simulink model "HIL_Testing_SW_amantest"  (Simulink 7.5)
settings: Solver=ode1  StartTime=0.0  StopTime=Inf  FixedStep=0.001  RelTol=1e-3
PostLoadFcn:
  | , if any(exist('dsrtsu_mdlpostloadfcn', 'file') == [2, 3, 6]), try dsrtsu_mdlpostloadfcn('Execute', bdroot); catch fprintf('Error in PostLoadFcn (dsrtsu_mdlpostloadfcn) for model "%s":\n %s\n', bdroot, lasterr); end, end,
undefined symbols (not defined in the file): CeBSER_Cnt_NumTempAxisPts, ChargeCord, ChargeCord_Control, ChargeToSOCCurr, ChrgCurrLim, CrntSens1Fine, CS_SOCSetPt, CyclerMaxChrgPwr, CyclerMaxDschrgPwr, deltaAhr, Drive_1, Drive_10, Drive_11, Drive_12, Drive_13, Drive_14, Drive_15, Drive_16, Drive_17, Drive_18, Drive_19, Drive_2, Drive_20, Drive_21, Drive_22, Drive_23, Drive_24, Drive_25, Drive_26, Drive_27, Drive_28, Drive_29, Drive_3, Drive_30, Drive_31, Drive_32, Drive_33, Drive_34, Drive_35, Drive_36, Drive_37, Drive_38, Drive_39, Drive_4, Drive_40, Drive_41, Drive_42, Drive_43, Drive_44, Drive_45, Drive_46, Drive_47, Drive_48, Drive_49, Drive_5, Drive_50, Drive_51, Drive_6, Drive_7, Drive_8 ... (+50)
libraries: simulink x129, rtican x50, rti2211sailib x5, rti2211serlib x5, rti2202miolib x3
(part 5 of 23)

== system HIL_Testing_SW_amantest/RX/Read EREV ==
  Enable : EnablePort
  Read HVEM : Subsystem
  Read PTEX : Subsystem
  LT_PwrDschLmt : Outport  OutDataType=sfix(16)  OutScaling=2^0
  LT_PwrChgLmt : Outport  Port=2  OutDataType=sfix(16)  OutScaling=2^0
  SOC : Outport  Port=3  OutDataType=sfix(16)  OutScaling=2^0
  SumOfCells : Outport  Port=4  OutDataType=sfix(16)  OutScaling=2^0
  MinCell : Outport  Port=5  OutDataType=sfix(16)  OutScaling=2^0
  MaxCell : Outport  Port=6  OutDataType=sfix(16)  OutScaling=2^0
  MinSectionVoltage : Outport  Port=7  OutDataType=sfix(16)  OutScaling=2^0
  HVCntctrStat : Outport  Port=8  OutDataType=sfix(16)  OutScaling=2^0
  PackCurrent : Outport  Port=9  OutDataType=sfix(16)  OutScaling=2^0
  PackVoltage : Outport  Port=10  OutDataType=sfix(16)  OutScaling=2^0
  BatTemp : Outport  Port=11  OutDataType=sfix(16)  OutScaling=2^0
  HVBatVltUpLmt_CAN : Outport  Port=12  OutDataType=sfix(16)  OutScaling=2^0
  HVBatVltLwLmt_CAN : Outport  Port=13  OutDataType=sfix(16)  OutScaling=2^0
  HVBatStOfChrgMin_CAN : Outport  Port=14  OutDataType=sfix(16)  OutScaling=2^0
  HVBatCrntLwLmt_CAN : Outport  Port=15  OutDataType=sfix(16)  OutScaling=2^0
  HVBatCrntUpLmt_CAN : Outport  Port=16  OutDataType=sfix(16)  OutScaling=2^0
  wires:
  Read PTEX/1(LT_PwrDschLmt) -> LT_PwrDschLmt/1
  Read PTEX/2(LT_PwrChgLmt) -> LT_PwrChgLmt/1
  Read PTEX/3(SOC) -> SOC/1
  Read HVEM/1(SumOfCells) -> SumOfCells/1
  Read HVEM/2(MinCell) -> MinCell/1
  Read HVEM/3(MaxCell) -> MaxCell/1
  Read HVEM/4(MinSectionVoltage) -> MinSectionVoltage/1
  Read HVEM/5(HVCntctrStat) -> HVCntctrStat/1
  Read HVEM/6(PackCurrent) -> PackCurrent/1
  Read HVEM/7(PackVoltage) -> PackVoltage/1
  Read HVEM/8(BatTemp) -> BatTemp/1
  Read PTEX/4(HVBatVltUpLmt_CAN) -> HVBatVltUpLmt_CAN/1
  Read PTEX/5(HVBatVltLwLmt_CAN) -> HVBatVltLwLmt_CAN/1
  Read PTEX/6(HVBatStOfChrgMin_CAN) -> HVBatStOfChrgMin_CAN/1
  Read PTEX/7(HVBatCrntLwLmt_CAN) -> HVBatCrntLwLmt_CAN/1
  Read PTEX/8(HVBatCrntUpLmt_CAN) -> HVBatCrntUpLmt_CAN/1

== system HIL_Testing_SW_amantest/TX/Chamber ==
  BatTemp : Inport  OutDataType=fixdt(1, 16)  OutScaling=2^0
  SetChamberT_ToBatTemp : Inport  Port=2  OutDataType=fixdt(1, 16)  OutScaling=2^0
  ChamberT_SwitchSlct : Subsystem  TreatAsAtomicUnit=on
  Multiport Switch : MultiPortSwitch  Inputs=39  zeroidx=off  OutDataTypeMode=uint8  OutDataType=fixdt(1, 16)  OutScaling=2^0  OutDataTypeStr=uint8
  SendTxToChamber : Subsystem  TreatAsAtomicUnit=on
  SetChamberTo10C : Constant  Value=[1 6 0 60 0 100 72 45]  OutDataTypeMode=uint8  OutDataType=fixdt(1, 16)  OutScaling=2^0  OutDataTypeStr=uint8
  SetChamberTo12p5C : Constant  Value=[1 6 0 60 0 125 137 231]  OutDataTypeMode=uint8  OutDataType=fixdt(1, 16)  OutScaling=2^0  OutDataTypeStr=uint8
  SetChamberTo15C : Constant  Value=[1 6 0 60 0 150 201 168]  OutDataTypeMode=uint8  OutDataType=fixdt(1, 16)  OutScaling=2^0  OutDataTypeStr=uint8
  SetChamberTo17p5C : Constant  Value=[1 6 0 60 0 175 9 186]  OutDataTypeMode=uint8  OutDataType=fixdt(1, 16)  OutScaling=2^0  OutDataTypeStr=uint8
  SetChamberTo20C : Constant  Value=[1 6 0 60 0 200 72 80]  OutDataTypeMode=uint8  OutDataType=fixdt(1, 16)  OutScaling=2^0  OutDataTypeStr=uint8
  SetChamberTo22p5C : Constant  Value=[1 6 0 60 0 225 137 142]  OutDataTypeMode=uint8  OutDataType=fixdt(1, 16)  OutScaling=2^0  OutDataTypeStr=uint8
  SetChamberTo25C : Constant  Value=[1 6 0 60 0 250 201 133]  OutDataTypeMode=uint8  OutDataType=fixdt(1, 16)  OutScaling=2^0  OutDataTypeStr=uint8
  SetChamberTo27p5C : Constant  Value=[1 6 0 60 1 19 9 155]  OutDataTypeMode=uint8  OutDataType=fixdt(1, 16)  OutScaling=2^0  OutDataTypeStr=uint8
  SetChamberTo2p5C : Constant  Value=[1 6 0 60 0 25 136 12]  OutDataTypeMode=uint8  OutDataType=fixdt(1, 16)  OutScaling=2^0  OutDataTypeStr=uint8
  SetChamberTo30C : Constant  Value=[1 6 0 60 1 44 73 139]  OutDataTypeMode=uint8  OutDataType=fixdt(1, 16)  OutScaling=2^0  OutDataTypeStr=uint8
  SetChamberTo32p5C : Constant  Value=[1 6 0 60 1 69 137 165]  OutDataTypeMode=uint8  OutDataType=fixdt(1, 16)  OutScaling=2^0  OutDataTypeStr=uint8
  SetChamberTo35C : Constant  Value=[1 6 0 60 1 94 201 174]  OutDataTypeMode=uint8  OutDataType=fixdt(1, 16)  OutScaling=2^0  OutDataTypeStr=uint8
  SetChamberTo37p5C : Constant  Value=[1 6 0 60 1 119 8 112]  OutDataTypeMode=uint8  OutDataType=fixdt(1, 16)  OutScaling=2^0  OutDataTypeStr=uint8
  SetChamberTo40C : Constant  Value=[1 6 0 60 1 144 72 58]  OutDataTypeMode=uint8  OutDataType=fixdt(1, 16)  OutScaling=2^0  OutDataTypeStr=uint8
  SetChamberTo42p5C : Constant  Value=[1 6 0 60 1 169 136 40]  OutDataTypeMode=uint8  OutDataType=fixdt(1, 16)  OutScaling=2^0  OutDataTypeStr=uint8
  SetChamberTo45C : Constant  Value=[1 6 0 60 1 194 201 199]  OutDataTypeMode=uint8  OutDataType=fixdt(1, 16)  OutScaling=2^0  OutDataTypeStr=uint8
  SetChamberTo47p5C : Constant  Value=[1 6 0 60 1 219 8 13]  OutDataTypeMode=uint8  OutDataType=fixdt(1, 16)  OutScaling=2^0  OutDataTypeStr=uint8
  SetChamberTo50C : Constant  Value=[1 6 0 60 1 244 73 209]  OutDataTypeMode=uint8  OutDataType=fixdt(1, 16)  OutScaling=2^0  OutDataTypeStr=uint8
  SetChamberTo52p5C : Constant  Value=[1 6 0 60 2 13 137 99]  OutDataTypeMode=uint8  OutDataType=fixdt(1, 16)  OutScaling=2^0  OutDataTypeStr=uint8
  SetChamberTo55C : Constant  Value=[1 6 0 60 2 38 201 124]  OutDataTypeMode=uint8  OutDataType=fixdt(1, 16)  OutScaling=2^0  OutDataTypeStr=uint8
  SetChamberTo57p5C : Constant  Value=[1 6 0 60 2 63 8 182]  OutDataTypeMode=uint8  OutDataType=fixdt(1, 16)  OutScaling=2^0  OutDataTypeStr=uint8
  SetChamberTo5C : Constant  Value=[1 6 0 60 0 50 200 19]  OutDataTypeMode=uint8  OutDataType=fixdt(1, 16)  OutScaling=2^0  OutDataTypeStr=uint8
  SetChamberTo60C : Constant  Value=[1 6 0 60 2 88 73 92]  OutDataTypeMode=uint8  OutDataType=fixdt(1, 16)  OutScaling=2^0  OutDataTypeStr=uint8
  SetChamberTo62p5C : Constant  Value=[1 6 0 60 2 113 136 130]  OutDataTypeMode=uint8  OutDataType=fixdt(1, 16)  OutScaling=2^0  OutDataTypeStr=uint8
  SetChamberTo65C : Constant  Value="[1 6 0 60 2  138 201 1]"  OutDataTypeMode=uint8  OutDataType=fixdt(1, 16)  OutScaling=2^0  OutDataTypeStr=uint8
  SetChamberTo7p5C : Constant  Value=[1 6 0 60 0 75 9 241]  OutDataTypeMode=uint8  OutDataType=fixdt(1, 16)  OutScaling=2^0  OutDataTypeStr=uint8
  SetChamberToMinus10C : Constant  Value=[1 6 0 60 255 156 8 95]  OutDataTypeMode=uint8  OutDataType=fixdt(1, 16)  OutScaling=2^0  OutDataTypeStr=uint8
  SetChamberToMinus12p5C : Constant  Value=[1 6 0 60 255 131 73 151]  OutDataTypeMode=uint8  OutDataType=fixdt(1, 16)  OutScaling=2^0  OutDataTypeStr=uint8
  SetChamberToMinus15C : Constant  Value=[1 6 0 60 255 106 136 25]  OutDataTypeMode=uint8  OutDataType=fixdt(1, 16)  OutScaling=2^0  OutDataTypeStr=uint8
  SetChamberToMinus17p5C : Constant  Value=[1 6 0 60 255 81 201 202]  OutDataTypeMode=uint8  OutDataType=fixdt(1, 16)  OutScaling=2^0  OutDataTypeStr=uint8
  SetChamberToMinus20C : Constant  Value=[1 6 0 60 255 56 9 228]  OutDataTypeMode=uint8  OutDataType=fixdt(1, 16)  OutScaling=2^0  OutDataTypeStr=uint8
  SetChamberToMinus22p5C : Constant  Value=[1 6 0 60 255 31 73 254]  OutDataTypeMode=uint8  OutDataType=fixdt(1, 16)  OutScaling=2^0  OutDataTypeStr=uint8
  SetChamberToMinus25C : Constant  Value=[1 6 0 60 255 6 136 52]  OutDataTypeMode=uint8  OutDataType=fixdt(1, 16)  OutScaling=2^0  OutDataTypeStr=uint8
  SetChamberToMinus27p5C : Constant  Value=[1 6 0 60 254 237 201 235]  OutDataTypeMode=uint8  OutDataType=fixdt(1, 16)  OutScaling=2^0  OutDataTypeStr=uint8
  SetChamberToMinus2p5C : Constant  Value=[1 6 0 60 255 231 72 124]  OutDataTypeMode=uint8  OutDataType=fixdt(1, 16)  OutScaling=2^0  OutDataTypeStr=uint8
  SetChamberToMinus30C : Constant  Value=[1 6 0 60 254 212 9 249]  OutDataTypeMode=uint8  OutDataType=fixdt(1, 16)  OutScaling=2^0  OutDataTypeStr=uint8
  SetChamberToMinus5C : Constant  Value=[1 6 0 60 255 206 137 162]  OutDataTypeMode=uint8  OutDataType=fixdt(1, 16)  OutScaling=2^0  OutDataTypeStr=uint8
  SetChamberToMinus7p5C : Constant  Value=[1 6 0 60 255 181 201 129]  OutDataTypeMode=uint8  OutDataType=fixdt(1, 16)  OutScaling=2^0  OutDataTypeStr=uint8
  SetChamberToZeroC : Constant  Value=[1 6 0 60 0 0 73 198]  OutDataTypeMode=uint8  OutDataType=fixdt(1, 16)  OutScaling=2^0  OutDataTypeStr=uint8
  Trigger_200ms : Subsystem  TreatAsAtomicUnit=on
      settings: CopyFcn=breaklink(gcb)
      mask Type: EnabledFunctionCall
      mask Description:
      | Execute a function-call subsystem at an inherited rate if enabled.
      | 
      | Demux the block's output to execute multiple function-call subsystems in a prescribed order.  The system connected to first demux port is executed first, the system connected to second demux port is executed second, and so on.
      mask Help: web(char(which([char(get_param(gcb,'MaskType')),'.html'])));
      mask Display: disp('f()')
  Trigger_200ms2 : Subsystem  TreatAsAtomicUnit=on
      settings: CopyFcn=breaklink(gcb)
      mask Type: EnabledFunctionCall
      mask Description:
      | Execute a function-call subsystem at an inherited rate if enabled.
      | 
      | Demux the block's output to execute multiple function-call subsystems in a prescribed order.  The system connected to first demux port is executed first, the system connected to second demux port is executed second, and so on.
      mask Help: web(char(which([char(get_param(gcb,'MaskType')),'.html'])));
      mask Display: disp('f()')
  wires:
  Multiport Switch/1 -> SendTxToChamber/1(ChamberTempCommand)
  Trigger_200ms2/1(Output Parameter) -> ChamberT_SwitchSlct/Trigger
  Trigger_200ms/1(Output Parameter) -> SendTxToChamber/Trigger  "TriggerMe"
  SetChamberToMinus30C/1 -> Multiport Switch/2
  SetChamberToMinus27p5C/1 -> Multiport Switch/3
  SetChamberToMinus25C/1 -> Multiport Switch/4
  SetChamberToMinus22p5C/1 -> Multiport Switch/5
  SetChamberToMinus20C/1 -> Multiport Switch/6
  SetChamberToMinus17p5C/1 -> Multiport Switch/7
  SetChamberToMinus15C/1 -> Multiport Switch/8
  SetChamberToMinus12p5C/1 -> Multiport Switch/9
  SetChamberToMinus10C/1 -> Multiport Switch/10
  SetChamberToMinus7p5C/1 -> Multiport Switch/11
  SetChamberToMinus5C/1 -> Multiport Switch/12
  SetChamberToMinus2p5C/1 -> Multiport Switch/13
  SetChamberToZeroC/1 -> Multiport Switch/14
  SetChamberTo2p5C/1 -> Multiport Switch/15
  SetChamberTo5C/1 -> Multiport Switch/16
  SetChamberTo7p5C/1 -> Multiport Switch/17
  SetChamberTo10C/1 -> Multiport Switch/18
  SetChamberTo12p5C/1 -> Multiport Switch/19
  SetChamberTo15C/1 -> Multiport Switch/20
  SetChamberTo17p5C/1 -> Multiport Switch/21
  SetChamberTo20C/1 -> Multiport Switch/22
  SetChamberTo22p5C/1 -> Multiport Switch/23
  SetChamberTo25C/1 -> Multiport Switch/24
  SetChamberTo27p5C/1 -> Multiport Switch/25
  SetChamberTo30C/1 -> Multiport Switch/26
  SetChamberTo32p5C/1 -> Multiport Switch/27
  SetChamberTo35C/1 -> Multiport Switch/28
  SetChamberTo37p5C/1 -> Multiport Switch/29
  SetChamberTo40C/1 -> Multiport Switch/30
  SetChamberTo42p5C/1 -> Multiport Switch/31
  SetChamberTo45C/1 -> Multiport Switch/32
  SetChamberTo47p5C/1 -> Multiport Switch/33
  SetChamberTo50C/1 -> Multiport Switch/34
  SetChamberTo52p5C/1 -> Multiport Switch/35
  SetChamberTo55C/1 -> Multiport Switch/36
  SetChamberTo57p5C/1 -> Multiport Switch/37
  SetChamberTo60C/1 -> Multiport Switch/38
  SetChamberTo62p5C/1 -> Multiport Switch/39
  SetChamberTo65C/1 -> Multiport Switch/40
  BatTemp/1 -> ChamberT_SwitchSlct/1(BatTemp)
  ChamberT_SwitchSlct/1(BatT_SwitchNumSlct) -> Multiport Switch/1
  SetChamberT_ToBatTemp/1 -> ChamberT_SwitchSlct/2(SetChamberT_ToBatTemp)

== system HIL_Testing_SW_amantest/TX/Chiller ==
  BatTemp : Inport  OutDataType=fixdt(1, 16)  OutScaling=2^0
  ContactorLine : Inport  Port=2  OutDataType=fixdt(1, 16)  OutScaling=2^0
  ProfileBatTemp : Inport  Port=3  OutDataType=fixdt(1, 16)  OutScaling=2^0
  BatTempOffset : Constant  OutDataTypeMode=single  OutDataType=fixdt(1, 16)  OutScaling=2^0  OutDataTypeStr=single
  ChillerCmndTxDecision : Subsystem  TreatAsAtomicUnit=on
  ChillerOpMode : Constant  OutDataTypeMode=uint8  OutDataType=fixdt(1, 16)  OutScaling=2^0  OutDataTypeStr=uint8
  Compare To Constant : simulink/Logic and Bit Operations/Compare To Constant  SystemSampleTime=-1  relop=~=  const=1  LogicOutDataTypeMode=boolean
  Compare To Constant1 : simulink/Logic and Bit Operations/Compare To Constant  SystemSampleTime=-1  relop===  const=3  LogicOutDataTypeMode=boolean
  ManualChillerPower : Constant  Value=0  OutDataTypeMode=boolean  OutDataType=fixdt(1, 16)  OutScaling=2^0  OutDataTypeStr=boolean  LockScale=on
  ManualChillerPower1 : Constant  OutDataTypeMode=boolean  OutDataType=fixdt(1, 16)  OutScaling=2^0  OutDataTypeStr=boolean  LockScale=on
  ManualChillerT_SP : Constant  Value=single(25.1)  OutDataType=fixdt(1, 16)  OutScaling=2^0
  Power1 : Constant  Value=0  OutDataTypeMode=boolean  OutDataType=fixdt(1, 16)  OutScaling=2^0  OutDataTypeStr=boolean
  Power2 : Constant  OutDataTypeMode=boolean  OutDataType=fixdt(1, 16)  OutScaling=2^0  OutDataTypeStr=boolean
  Sum : Sum  OutDataType=fixdt(1, 16)  OutScaling=2^0
  Switch : Switch  Threshold=0.5  OutDataType=fixdt(1, 16)  OutScaling=2^0
  Switch1 : Switch  Threshold=0.5  OutDataType=fixdt(1, 16)  OutScaling=2^0
  Switch2 : Switch  Threshold=0.5  OutDataType=fixdt(1, 16)  OutScaling=2^0
  Trigger_200ms1 : Subsystem  TreatAsAtomicUnit=on
      settings: CopyFcn=breaklink(gcb)
      mask Type: EnabledFunctionCall
      mask Description:
      | Execute a function-call subsystem at an inherited rate if enabled.
      | 
      | Demux the block's output to execute multiple function-call subsystems in a prescribed order.  The system connected to first demux port is executed first, the system connected to second demux port is executed second, and so on.
      mask Help: web(char(which([char(get_param(gcb,'MaskType')),'.html'])));
      mask Display: disp('f()')
  wires:
  ContactorLine/1 -> Switch/2
  Power1/1 -> Switch/3
  Power2/1 -> Switch/1
  Switch/1 -> ChillerCmndTxDecision/2(ChillerOnOff)  "ChillerOnOff"
  Trigger_200ms1/1(Output Parameter) -> ChillerCmndTxDecision/Trigger
  ChillerOpMode/1 -> ChillerCmndTxDecision/3(ChillerOpMode), [ChillerOpMode]  "ChillerOpMode"
  ManualChillerPower/1 -> Switch1/3  "ManualChillerPower"
  Compare To Constant/1 -> Switch1/2
  ManualChillerPower1/1 -> Switch1/1
  [ChillerOpMode] -> Compare To Constant/1
  Switch1/1 -> ChillerCmndTxDecision/5(ManualChillerPower)
  ProfileBatTemp/1 -> Switch2/1  "ProfileBatTemp"
  ManualChillerT_SP/1 -> Switch2/3  "ManualChillerT_SP"
  [ChillerOpMode] -> Compare To Constant1/1
  Compare To Constant1/1 -> Switch2/2
  Switch2/1 -> ChillerCmndTxDecision/4(ChillerT_SP)
  BatTempOffset/1 -> Sum/2
  BatTemp/1 -> Sum/1
  Sum/1 -> ChillerCmndTxDecision/1(BatTemp)

== system HIL_Testing_SW_amantest/TX/PrpslnAtv ==
  ContactorLine : Inport  OutDataType=fixdt(1, 16)  OutScaling=2^0
  Active : Constant  OutDataTypeMode=boolean  OutDataType=fixdt(1, 16)  OutScaling=2^0  OutDataTypeStr=boolean
  DriveSelect3 : Switch  Threshold=0.5  OutDataTypeMode=double  OutDataType=fixdt(1, 16)  OutScaling=2^0  OutDataTypeStr=double
  Function-Call Generator : simulink/Ports & Subsystems/Function-Call Generator  sample_time=0.025  numberOfIterations=1
  Off : Constant  Value=0  OutDataTypeMode=boolean  OutDataType=fixdt(1, 16)  OutScaling=2^0  OutDataTypeStr=boolean
  msg_0x1DF_3e9_1F1 : Subsystem  Tag=x.x
      mask Type: Subsystem
      mask Display:
      | text(.52,.01,char(get_param(gcb,'Tag') ), 'horizontalAlignment','center','verticalAlignment','bottom' )
      | disp(get_param(gcb,'Name'))
  wires:
  DriveSelect3/1 -> msg_0x1DF_3e9_1F1/1(PrplsnAtv)
  Active/1 -> DriveSelect3/1
  Off/1 -> DriveSelect3/3
  ContactorLine/1 -> DriveSelect3/2
  Function-Call Generator/1 -> [Trigg_25ms]
  [Trigg_25ms] -> msg_0x1DF_3e9_1F1/Trigger

== system HIL_Testing_SW_amantest/TX/TX PTEI ==
  BatVolt : Inport  OutDataType=fixdt(1, 16)  OutScaling=2^0
  Ignition : Inport  Port=2  OutDataType=fixdt(1, 16)  OutScaling=2^0
  ContactorLine : Inport  Port=3  OutDataType=fixdt(1, 16)  OutScaling=2^0
  Transfer Fcn : TransferFcn  Denominator=[.085 1]
  Tx_Contactor_Msg : Subsystem
  wires:
  Transfer Fcn/1 -> Tx_Contactor_Msg/1(HVInvRatVlt)
  BatVolt/1 -> Transfer Fcn/1, Tx_Contactor_Msg/2(BatteryVoltage)
  Ignition/1 -> Tx_Contactor_Msg/3(Ignition)
  ContactorLine/1 -> Tx_Contactor_Msg/4(ContactorLine)

== system HIL_Testing_SW_amantest/TX/Tx_Cycler ==
  Control_Value_Proc : Inport  OutDataType=sfix(16)  OutScaling=2^0
  Control_Mode : Inport  Port=2  OutDataType=sfix(16)  OutScaling=2^0
  Version_Number : Inport  Port=3  OutDataType=sfix(16)  OutScaling=2^0
  Hardware_Version : Inport  Port=4  OutDataType=sfix(16)  OutScaling=2^0
  Rx_status : Inport  Port=5  OutDataType=sfix(16)  OutScaling=2^0
  Converter_Status_B : Inport  Port=6  OutDataType=sfix(16)  OutScaling=2^0
  StationID_B1 : Inport  Port=7  OutDataType=sfix(16)  OutScaling=2^0
  StationID_B : Inport  Port=8  OutDataType=sfix(16)  OutScaling=2^0
  Bus Creator1 : BusCreator  Inputs=3
  Data Store Read{,1..4} (5 alike) : DataStoreRead  DataStoreName=Channel  SampleTime=0
  Data Store Read5 : DataStoreRead  DataStoreName=Handshake  SampleTime=0
  Data Store Read6 : DataStoreRead  DataStoreName=LocalModeRequest  SampleTime=0
  Data Type Conversion : DataTypeConversion  OutDataTypeMode=boolean  OutDataType=fixdt(1, 16)  OutScaling=2^0  OutDataTypeStr=boolean
  Data Type Conversion1 : DataTypeConversion  OutDataTypeMode=boolean  OutDataType=fixdt(1, 16)  OutScaling=2^0  OutDataTypeStr=boolean
  Detect Increase : simulink/Logic and Bit Operations/Detect Increase  SystemSampleTime=-1  vinit=0.0
  Detect Increase1 : simulink/Logic and Bit Operations/Detect Increase  SystemSampleTime=-1  vinit=0.0
  Logical Operator{1,3..5} (4 alike) : Logic  AllPortsSameDT=off  OutDataTypeMode=boolean  OutDataTypeStr=boolean
  Logical Operator2 : Logic  Operator=NOT  AllPortsSameDT=off  OutDataTypeMode=boolean  LogicDataType=fixdt(0, 8)  OutDataTypeStr=boolean
  Logical Operator6 : Logic  Operator=NOT  AllPortsSameDT=off  OutDataTypeMode=boolean  LogicDataType=fixdt(0, 8)  OutDataTypeStr=boolean
  Send Greeting : Subsystem  TreatAsAtomicUnit=on
  Send Ping : Subsystem  TreatAsAtomicUnit=on
  Send Remote Request A : Subsystem  TreatAsAtomicUnit=on
  Send Remote Request B : Subsystem  TreatAsAtomicUnit=on
  Subsystem : Subsystem
  TX_ABC_ChA : Subsystem  TreatAsAtomicUnit=on
  TX_ABC_ChB : Subsystem  TreatAsAtomicUnit=on
  Take_Cycler_Command : Stateflow chart  TreatAsAtomicUnit=on
  wires:
  Version_Number/1 -> Take_Cycler_Command/1(Version), [Version_Number]
  Rx_status/1 -> Subsystem/1(In)
  Converter_Status_B/1 -> Take_Cycler_Command/4(Side_B_Status)
  Detect Increase/1 -> Data Type Conversion/1
  Take_Cycler_Command/1(Send_Ping) -> Send Ping/Enable
  Take_Cycler_Command/2(Send_Greeting) -> Send Greeting/Enable
  Take_Cycler_Command/4(Channel_Change_B) -> Bus Creator1/1
  Take_Cycler_Command/5(Control_From_B) -> Bus Creator1/2
  Take_Cycler_Command/6(Control_To_B) -> Bus Creator1/3
  Subsystem/1(Out) -> Take_Cycler_Command/3(Status)
  Detect Increase1/1 -> Data Type Conversion1/1
  Hardware_Version/1 -> [Hardware_Version]
  [Hardware_Version] -> Take_Cycler_Command/2(Hardware)
  [Hardware_Version] -> Send Remote Request A/4(Hardware_Version)
  [Hardware_Version] -> Send Greeting/2(Hardware)
  [Version_Number] -> Send Greeting/1(Version)
  Data Type Conversion/1 -> Take_Cycler_Command/5(Perform_Handshake)
  Data Type Conversion1/1 -> Take_Cycler_Command/6(Reset_to_Local)
  Data Store Read/1 -> Take_Cycler_Command/7(Channel)
  Take_Cycler_Command/7(Send_Commands) -> [Send_Commands]
  [Send_Commands] -> Logical Operator3/2
  Data Store Read1/1 -> Logical Operator2/1
  Logical Operator2/1 -> Logical Operator3/1
  Logical Operator3/1 -> TX_ABC_ChA/Enable
  [Control_Value_Proc] -> TX_ABC_ChA/1(Control_Value)
  [Control_Mode] -> TX_ABC_ChA/2(Control_Mode)
  [Send_Commands] -> Logical Operator1/2
  Data Store Read2/1 -> Logical Operator1/1
  Logical Operator1/1 -> TX_ABC_ChB/Enable
  [Control_Value_Proc] -> TX_ABC_ChB/1(Control_Value)
  [Control_Mode] -> TX_ABC_ChB/2(Control_Mode)
  Take_Cycler_Command/3(Send_Remote_Req_B) -> [RemoteRequest]
  [RemoteRequest] -> Logical Operator4/1
  Logical Operator4/1 -> Send Remote Request A/Enable
  Logical Operator5/1 -> Send Remote Request B/Enable
  Data Store Read3/1 -> Logical Operator6/1
  Logical Operator6/1 -> Logical Operator4/2
  [RemoteRequest] -> Logical Operator5/1
  Data Store Read4/1 -> Logical Operator5/2
  [StationID_X1] -> Send Remote Request A/2(StationID_B1)
  [StationID_X1] -> Send Remote Request B/2(StationID_B1)
  [StationID_X] -> Send Remote Request B/3(StationID_B)
  [StationID_X] -> Send Remote Request A/3(StationID_B)
  [Hardware_Version] -> Send Remote Request B/4(Hardware_Version)
  Bus Creator1/1 -> [Control]
  [Control] -> Send Remote Request B/1(Control)
  [Control] -> Send Remote Request A/1(Control)
  Data Store Read5/1 -> Detect Increase/1
  Data Store Read6/1 -> Detect Increase1/1
  Control_Value_Proc/1 -> [Control_Value_Proc]
  Control_Mode/1 -> [Control_Mode]
  StationID_B1/1 -> [StationID_X1]
  StationID_B/1 -> [StationID_X]

== system HIL_Testing_SW_amantest/HWO/TX HVEM/ChargeCord_Control ==
  ChrgCordConnect : Inport  OutDataType=sfix(16)  OutScaling=2^0
  110V : Inport  Port=2  OutDataType=sfix(16)  OutScaling=2^0
  220V : Inport  Port=3  OutDataType=sfix(16)  OutScaling=2^0
  None : Inport  Port=4  OutDataType=sfix(16)  OutScaling=2^0
  HVChrgACEnStat : Inport  Port=5  OutDataType=sfix(16)  OutScaling=2^0
  110 : Subsystem  TreatAsAtomicUnit=on
  220 : Subsystem  TreatAsAtomicUnit=on
  Connected_Freq : Constant  Value=1000  OutDataTypeMode=uint32  OutDataType=sfix(16)  OutScaling=2^0  OutDataTypeStr=uint32
  Connected_PrcsdVoltFreq : Constant  Value=1000  OutDataTypeMode=uint32  OutDataType=sfix(16)  OutScaling=2^0  OutDataTypeStr=uint32
  Connected_Prox : Constant  Value=1.6  OutDataType=sfix(16)  OutScaling=2^0  OutDataTypeStr=Inherit: Inherit via back propagation
  Cord Connected : Subsystem  TreatAsAtomicUnit=on
      settings: PropExecContextOutsideSubsystem=on
  Cord Not Connected : Subsystem  TreatAsAtomicUnit=on
  Data Type Conversion : DataTypeConversion  OutDataType=sfix(16)  OutScaling=2^0
  Data Type Conversion1 : DataTypeConversion  OutDataType=sfix(16)  OutScaling=2^0
  Data Type Conversion2 : DataTypeConversion  OutDataType=sfix(16)  OutScaling=2^0
  Disconnected : Subsystem  TreatAsAtomicUnit=on
  If : If  IfExpression=u1 ~= 0  ZeroCross=off
  If1 : If  NumInputs=2  IfExpression=u1==1  ElseIfExpressions=u2==1  ZeroCross=off
  Logical Operator1 : Logic  Operator=OR  AllPortsSameDT=off  OutDataTypeMode=boolean  OutDataTypeStr=boolean
  Logical Operator2 : Logic  Operator=OR  AllPortsSameDT=off  OutDataTypeMode=boolean  OutDataTypeStr=boolean
  Merge{,1..4,6..8} (8 alike) : Merge
  Merge5 : Merge  Inputs=3
  No Proximity : Constant  Value=0  OutDataType=sfix(16)  OutScaling=2^0  OutDataTypeStr=Inherit: Inherit via back propagation
  NotConnected_Current : Constant  Value=0  OutDataType=sfix(16)  OutScaling=2^0  OutDataTypeStr=Inherit: Inherit via back propagation
  NotConnected_DC : Constant  Value=0  OutDataType=sfix(16)  OutScaling=2^0  OutDataTypeStr=Inherit: Inherit via back propagation
  NotConnected_DC1 : Constant  Value=10  OutDataType=sfix(16)  OutScaling=2^0  OutDataTypeStr=Inherit: Inherit via back propagation
  NotConnected_Freq : Constant  Value=0  OutDataType=sfix(16)  OutScaling=2^0  OutDataTypeStr=Inherit: Inherit via back propagation
  NotConnected_Freq1 : Constant  Value=1000  OutDataType=sfix(16)  OutScaling=2^0  OutDataTypeStr=Inherit: Inherit via back propagation
  NotConnected_Temp : Constant  Value=0  OutDataType=sfix(16)  OutScaling=2^0  OutDataTypeStr=Inherit: Inherit via back propagation
  NotConnected_Voltage : Constant  Value=0  OutDataType=sfix(16)  OutScaling=2^0  OutDataTypeStr=Inherit: Inherit via back propagation
  OurLatchReset : Subsystem
  OurLatchReset1 : Subsystem
  Ve_OP_DC_ControlPilot : Outport  OutDataType=sfix(16)  OutScaling=2^0
  Ve_OP_t_ControlPilot_ms : Outport  Port=2  OutDataType=sfix(16)  OutScaling=2^0
  Proximity : Outport  Port=3  OutDataType=sfix(16)  OutScaling=2^0
  Voltage : Outport  Port=4  OutDataType=sfix(16)  OutScaling=2^0
  Current : Outport  Port=5  OutDataType=sfix(16)  OutScaling=2^0
  Temp : Outport  Port=6  OutDataType=sfix(16)  OutScaling=2^0
  PrcsdVolt_DC : Outport  Port=7  OutDataType=sfix(16)  OutScaling=2^0
  PrcsdVolt_Freq : Outport  Port=8  OutDataType=sfix(16)  OutScaling=2^0
  wires:
  Cord Not Connected/6(Temp) -> Merge8/2
  Cord Not Connected/5(Current) -> Merge7/2
  Cord Not Connected/4(Voltage) -> Merge6/2
  Cord Not Connected/3(Freq) -> Merge2/2
  Cord Not Connected/2(DC_out) -> Merge1/2
  Cord Not Connected/1(ChargeCrdPresent) -> Merge/2
  NotConnected_Temp/1 -> Cord Not Connected/6(Temp_in)
  NotConnected_Current/1 -> Cord Not Connected/5(Current_in)
  NotConnected_Voltage/1 -> Cord Not Connected/4(Voltage_in)
  NotConnected_Freq/1 -> Cord Not Connected/3(Freq_in)
  NotConnected_DC/1 -> Cord Not Connected/2(DC_in)
  No Proximity/1 -> Cord Not Connected/1(Proximity)
  [OutletType] -> Cord Connected/4(Outlet Type)
  Merge5/1 -> [OutletType]
  HVChrgACEnStat/1 -> Cord Connected/3(AC_Enable)
  Cord Connected/1(ChargeCrdPresent) -> Merge/1
  Merge/1 -> Proximity/1
  Connected_Prox/1 -> Cord Connected/1(Proximity)
  Merge1/1 -> Ve_OP_DC_ControlPilot/1
  Merge2/1 -> Ve_OP_t_ControlPilot_ms/1
  Connected_Freq/1 -> Cord Connected/2(Freq1)
  If/1 -> Cord Connected/Action
  If/2 -> Cord Not Connected/Action
  Cord Connected/2(DC) -> Merge1/1
  Cord Connected/3(Freq) -> Merge2/1
  110V/1 -> Data Type Conversion/1
  220V/1 -> Data Type Conversion2/1
  OurLatchReset/1(Out1) -> If1/1
  OurLatchReset1/1(Out1) -> If1/2
  If1/1 -> 110/Action
  If1/2 -> 220/Action
  If1/3 -> Disconnected/Action
  110/1(Out1) -> Merge5/1
  220/1(Out1) -> Merge5/2
  Disconnected/1(Out1) -> Merge5/3
  Logical Operator2/1 -> OurLatchReset/2(Reset)
  None/1 -> Data Type Conversion1/1
  Logical Operator1/1 -> OurLatchReset1/2(Reset)
  ChrgCordConnect/1 -> If/1
  Cord Connected/4(Voltage) -> Merge6/1
  Cord Connected/5(Current) -> Merge7/1
  Cord Connected/6(Temp) -> Merge8/1
  Merge8/1 -> Temp/1
  Merge7/1 -> Current/1
  Merge6/1 -> Voltage/1
  Data Type Conversion/1 -> Logical Operator1/2, OurLatchReset/1(U)
  Data Type Conversion1/1 -> Logical Operator1/1, Logical Operator2/1
  Data Type Conversion2/1 -> Logical Operator2/2, OurLatchReset1/1(U)
  Connected_PrcsdVoltFreq/1 -> Cord Connected/5(PrcsdVolt_Freq1)
  Cord Not Connected/7(PrcsdVolt_DC) -> Merge3/2
  Cord Not Connected/8(PrcsdVolt_Freq) -> Merge4/2
  Cord Connected/7(PrcsdVolt_DC) -> Merge3/1
  Cord Connected/8(PrcsdVolt_Freq) -> Merge4/1
  Merge3/1 -> PrcsdVolt_DC/1
  Merge4/1 -> PrcsdVolt_Freq/1
  NotConnected_DC1/1 -> Cord Not Connected/7(PrcsdVolt_DC_in)
  NotConnected_Freq1/1 -> Cord Not Connected/8(PrcsdVolt_Freq_in)

== system HIL_Testing_SW_amantest/HWO/TX HVEM/Trigger_25ms1 ==
  Function-Call Generator : simulink/Ports & Subsystems/Function-Call Generator  sample_time=0.025  numberOfIterations=1
  Output Parameter : Outport  OutDataType=sfix(16)  OutScaling=2^0
  wires:
  Function-Call Generator/1 -> Output Parameter/1
